simulink model "simulink_test"  (Simulink 7.9)
settings: Solver=ode45  StartTime=0.0  StopTime=10000  RelTol=1e-3
libraries: simulink x2
settings Model: Creator=atp10lbr  LastModifiedBy=atp10lbr

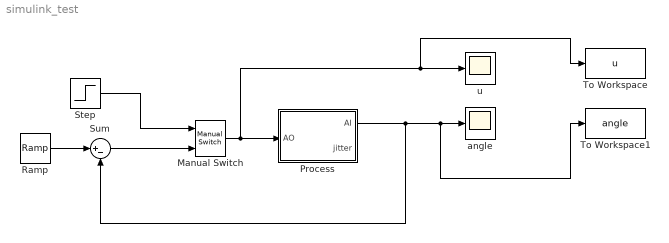
== system simulink_test ==
  Manual Switch : simulink/Signal Routing/Manual Switch  sw=1  action=0  varsize=off
  "Process " : Subsystem  mask(SISO Process){AOno=0, AIno=0, h=0.01}
      mask prompts: AOno "AO connection"; AIno "AI connection"; h "Sample Period"
      mask help:
      | Process communication block.
      | For use with Linux on PC with I/O.
      mask Help:
      | AO connection - specifies the analogue output connection on the I/O module on the back of the PC.
      | <p>
      | AI connection - specifies the analogue input connection on the I/O module on the back of the PC.
      | 
      | <p>
      |  Sample period - the sample period.
      | <p>
      | Jitter - vector with computer CPU load during sample periods, which ranges from zero to one. If value equal to one it is likely that a sample has been missed.
  Ramp : simulink/Sources/Ramp  slope=0.1  start=10  X0=-5
  Step : Step  Time=3  Before=-1  SampleTime=0
  Sum : Sum  Inputs=|+-
  To Workspace : ToWorkspace  VariableName=u  SampleTime=-1  SaveFormat=Timeseries
  To Workspace1 : ToWorkspace  VariableName=angle  SampleTime=-1  SaveFormat=Timeseries
  angle : Scope
      settings: TimeRange=200  YMin=-10  YMax=7.5
  u : Scope
      settings: TimeRange=200  YMin=-7  YMax=4
  wires:
  Ramp/1 -> Sum/1
  "Process "/1(AI) -> Sum/2, angle/1, To Workspace1/1
  Manual Switch/1 -> "Process "/1(AO), u/1, To Workspace/1
  Sum/1 -> Manual Switch/2
  Step/1 -> Manual Switch/1

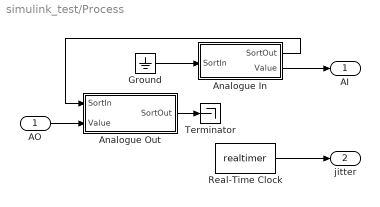
== system simulink_test/Process  ==
  AO : Inport
  Analogue In : Subsystem  mask(AnalogueIOBlock){h=h, AIno=AIno}
      mask prompts: h "Sample period"; AIno "Input port number"
      mask help: Analogue input block for use on PC running Linux.
  Analogue Out : Subsystem  mask(AnalogueIOBlock){h=h, AOno=AOno}
      mask prompts: h "Sample period"; AOno "Output port number"
      mask help: Analogue output block for use on PC running Linux
  Ground : Ground
  Real-Time Clock : S-Function  FunctionName=realtimer  Parameters=h  EnableBusSupport=off
  Terminator : Terminator
  AI : Outport  InitialOutput=0
  jitter : Outport  Port=2
  wires:
  Ground/1 -> Analogue In/1(SortIn)
  Analogue In/2(Value) -> AI/1
  Real-Time Clock/1 -> jitter/1
  AO/1 -> Analogue Out/2(Value)
  Analogue In/1(SortOut) -> Analogue Out/1(SortIn)
  Analogue Out/1(SortOut) -> Terminator/1

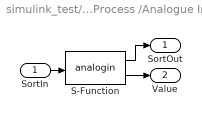
== system simulink_test/Process /Analogue In ==
  SortIn : Inport
  S-Function : S-Function  FunctionName=analogin  Parameters=h AIno  EnableBusSupport=off
  SortOut : Outport  InitialOutput=0
  Value : Outport  Port=2  InitialOutput=0
  wires:
  S-Function/2 -> Value/1
  SortIn/1 -> S-Function/1
  S-Function/1 -> SortOut/1

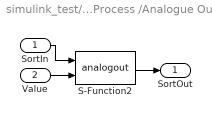
== system simulink_test/Process /Analogue Out ==
  SortIn : Inport
  Value : Inport  Port=2
  S-Function2 : S-Function  FunctionName=analogout  Parameters=h AOno  EnableBusSupport=off
  SortOut : Outport  InitialOutput=0
  wires:
  Value/1 -> S-Function2/2
  S-Function2/1 -> SortOut/1
  SortIn/1 -> S-Function2/1
